simulink library "sf_elevator_lib"  (Simulink 7.6)
settings: Solver=FixedStepDiscrete  StartTime=0.0  StopTime=10.0  FixedStep=1  RelTol=1e-3
settings Model: Creator=The MathWorks Inc.

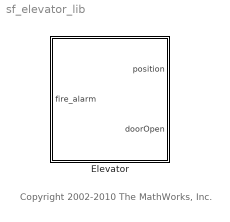
== system sf_elevator_lib ==
  note: Copyright 2002-2010 The MathWorks, Inc.
  Elevator : Stateflow chart  TreatAsAtomicUnit=on

== stateflow chart Elevator ==
  state dequeue(task_floor) [function]
    (junction 19) -> (junction 18) [order 2]
    (junction 19) -> (junction 20) [order 1] : [i < NUM_FLOOR]
    (junction 20) -> (junction 19) : {task_queue[i] = task_queue[i+1]; i++;}
    (junction 22) -> (junction 20) [order 2]
    (junction 22) -> (junction 21) [order 1] : [i >= NUM_FLOOR || task_queue[i] == 0]
    (junction 23) -> (junction 22) [order 2]
    (junction 23) -> (junction 23) [order 1] : [task_queue[i] > 0 && ...
        | i<NUM_FLOOR && ...
        | task_queue[i] != task_floor]{i++;}
    (default) -> (junction 23) : {i=0;}
  state PickUpDropOff
    en: Main_deregister(cur_floor);
    deregister(cur_floor);
    direction = MOVE_IDLE;
    doorOpen = 1;
    du: Main_deregister(cur_floor);
    deregister(cur_floor);
    ex: doorOpen = 0;
    state Stopped
    Stopped -> Stopped [order 2] : [fire_alarm]{status = EMERG;}
        | /* Resets the timeout counter */
  state Idle
    en: status = IDLE;
    ex: status = BUSY;
  state MoveToTask
    du: move_to(task_queue[0]);
  state move_to(destination) [function]
    (junction 30) -> (junction 27) [order 2]
    (junction 29) -> (junction 28) : {
        | /* Move down */
        | position = position - VELOCITY;
        | direction = MOVE_DOWN;
        | }
    (junction 30) -> (junction 29) [order 1] : [!move_up && move_down]
    (junction 33) -> (junction 30) [order 2]
    (junction 32) -> (junction 31) : {
        | /* Move up */
        | position = position + VELOCITY;
        | direction = MOVE_UP;
        | }
    (junction 33) -> (junction 32) [order 1] : [move_up && !move_down]
    (junction 34) -> (junction 33) : {
        | /* Move down */
        | move_down = (position - destination > ERR_TOR);
        | }
    (junction 35) -> (junction 34) : {
        | /* Move up */
        | move_up = (destination - position > ERR_TOR);
        | }
    (default) -> (junction 35)
  state ans = should_stop [function]
    (default) -> (junction 45)
    (junction 45) -> (junction 46) : {
        | /* 'INIT':Initialization */
        | cur_floor = ml_round(position);
        | }
    (junction 46) -> (junction 47) : {
        | /* Arrived destination */
        | at_destination = (fabs(position - task_queue[0]) < ERR_TOR);
        | }
    (junction 47) -> (junction 48) : {
        | /* Arrived at a floor */
        | at_a_floor = (fabs(position - cur_floor) < ERR_TOR);
        | }
    (junction 48) -> (junction 49) : {
        | /* There is car call to stop at this floor */
        | request_from_car = (car_call_status[cur_floor]);
        | }
    (junction 49) -> (junction 50) : {
        | /* There is hall call from this floor */
        | request_from_hall = (hall_call_status[cur_floor]);
        | }
    (junction 50) -> (junction 51) : {
        | /* This hall call is still outstanding in queue */
        | this_hall_call_outstanding = (Main_exists_in_queue(cur_floor));
        | }
    (junction 51) -> (junction 52) [order 1] : [at_destination]
    (junction 52) -> (junction 53) : {
        | /* 'S':Should stop at this floor */
        | position = cur_floor; /* Adjust position */
        | ans = 1;
        | }
    (junction 51) -> (junction 54) [order 2]
    (junction 54) -> (junction 55) [order 1] : [!at_a_floor]
    (junction 55) -> (junction 56) : {
        | /* 'C':Should not stop, continue */
        | ans = 0;
        | }
    (junction 54) -> (junction 57) [order 2]
    (junction 57) -> (junction 58) [order 1] : [request_from_car]
    (junction 58) -> (junction 59) : {
        | /* 'S':Should stop at this floor */
        | position = cur_floor; /* Adjust position */
        | ans = 1;
        | }
    (junction 57) -> (junction 60) [order 2]
    (junction 60) -> (junction 61) [order 1] : [request_from_hall && this_hall_call_outstanding]
    (junction 61) -> (junction 62) : {
        | /* 'S':Should stop at this floor */
        | position = cur_floor; /* Adjust position */
        | ans = 1;
        | }
    (junction 60) -> (junction 63) [order 2]
    (junction 63) -> (junction 64) : /* Default */
    (junction 64) -> (junction 65) : {
        | /* 'C':Should not stop, continue */
        | ans = 0;
        | }
  state dir = get_direction [function]
    (default) -> (junction 44) : {dir = direction;}
  state register(car_call_floor) [function]
    (default) -> (junction 43) : {enqueue(car_call_floor);
        | car_call_status[car_call_floor] = 1;}
  state enqueue(task_floor) [function]
    (junction 38) -> (junction 36) [order 2] : {task_queue[i] = task_floor;}
    (junction 38) -> (junction 37) [order 1] : [i >= NUM_FLOOR]
    (junction 39) -> (junction 38) [order 3]
    (junction 39) -> (junction 39) [order 2] : [task_queue[i] > 0 && i<NUM_FLOOR]{i++;}
    (junction 39) -> (junction 40) [order 1] : [task_queue[i] == task_floor]
    (junction 42) -> (junction 39) [order 2] : {i = 0;}
    (junction 42) -> (junction 41) [order 1] : [car_call_status[task_floor] != 0]
    (default) -> (junction 42)
  state pos = get_position [function]
    (default) -> (junction 26) : {pos = position;}
  state deregister(car_call_floor) [function]
    (default) -> (junction 25) : {dequeue(car_call_floor);
        | car_call_status[car_call_floor] = 0;}
  state stat = get_status [function]
    (default) -> (junction 24) : {stat = status;}
  (default) -> Idle : {doorOpen = 0;}
  (junction 17) -> Idle [order 2]
  Stopped -> (junction 17) [order 1] : after(TIME_OUT, sec)
  (junction 17) -> MoveToTask [order 1] : [task_queue[0]]
  Idle -> MoveToTask : [task_queue[0]]
  MoveToTask -> PickUpDropOff : [should_stop()]
  data: i temporary uint8; task_floor function_input uint8; destination function_input double; move_up temporary boolean =0; move_down temporary boolean =0; ans function_output boolean; at_destination temporary boolean =0; at_a_floor temporary boolean =0; request_from_car temporary boolean =0; request_from_hall temporary boolean =0; this_hall_call_outstanding temporary boolean =0; dir function_output uint8; car_call_floor function_input uint8; task_floor function_input uint8; i temporary uint8; pos function_output double; car_call_floor function_input uint8; stat function_output uint8; inputVal function_input double; out function_output double; VELOCITY constant double =0.005; NUM_FLOOR constant uint8 =9; ERR_TOR constant double =0.001; fire_alarm input boolean; TIME_OUT constant uint32 =1000; status local Enum: ElevatorStatus =ElevatorStatus.IDLE; position output double =1; task_queue local uint8 size=10; car_call_status local uint8 size=10; direction local Enum: ElevatorDirection =ElevatorDirection.MOVE_IDLE; doorOpen output boolean; cur_floor local uint8; hall_call_status data_store_memory double
  data move_up settings: description=Move up
  data move_down settings: description=Move down
  data at_destination settings: description=Arrived destination
  data at_a_floor settings: description=Arrived at a floor
  data request_from_car settings: description=There is car call to stop at this floor
  data request_from_hall settings: description=There is hall call from this floor
  data this_hall_call_outstanding settings: description=This hall call is still outstanding in queue
  function out = ml_round(inputVal):
    | function out = ml_round(inputVal)
    | 
    | out = round(inputVal);
